simulink model "BatteryEstim3RC_PTBS_v1"  (R2021b)
settings: Solver=ode45  StartTime=0.0  StopTime=3600*100  MaxStep=60  RelTol=1e-3
values from neighbouring files (symbols this model uses):
  CapacityAh = 18.45078888    [CRM_test2.mat]    (also in test_experimentalData.m = p(1,j))
  Em = [45.6901270717 46.4315814068 47.300952453 47.7790115007 48.2148195515 48.8978968293 49.5654324772 50.1873261848 50.9421309599 51.6669224049 52.4024883901 52.7506387312]    [CRM_test2.mat]
  InitialCapVoltage = [0 0 0]    [CRM_test2.mat]
  InitialChargeDeficitAh = 0    [CRM_test2.mat]    (also in test_experimentalData.m = p(2,j)*(1-SOC_0)*CapacityAh)
  R0 = [0.0235875392162 0.0245006787976 0.0256331806458 0.0242487665052 0.028405652821 0.0253523326352 0.028201644819 0.0293858743062 0.0295795385449 0.0307165268423 0.0287680896969 0.030864537146]    [CRM_test2.mat]
  Rx = [0.00541138390772 0.0212793802998 0.00233398938792 0.00525131200495 0.0214750772641 0.0118054508147 0.0052795280688 0.0206172338661 0.0267100492405 0.00529937987512 0.0207294874529 0.0276908855018 ... (36 elements, 3x12)]    [CRM_test2.mat]
  SOC_LUT = [0 0.19733502907 0.397240705949 0.465830267524 0.533618770668 0.604063407396 0.674817039043 0.746547331368 0.819156363357 0.892985414724 0.969511183307 1]    [CRM_test2.mat]
  Tx = [2.08733276285 29.8288343735 111.456817188 2.91727865649 28.0237475362 580.71656132 2.8704763749 27.9272337783 507.228077533 2.8038263246 29.292039832 509.28251447 ... (36 elements, 3x12)]    [CRM_test2.mat]
libraries: autolibbatterycommon x1
settings Model: ModifiedByFormat=The MathWorks, Inc.  Creator=The MathWorks, Inc.  LastModifiedBy=The MathWorks, Inc.
settings SolverCC: AlgebraicLoopSolver=TrustRegion
settings DataIOCC: ExternalInput=[psObj.Time, psObj.Current]  LoadExternalInput=on  SaveOutput=off  DSMLogging=off  SaveTime=off  ReturnWorkspaceOutputs=off
settings DebuggingCC: SFMachineParentedDataDiag=warning  ArithmeticOperatorsInVariantConditions=warning
settings SFSimCC: SimUseLocalCustomCode=off  CustomCodeUndefinedFunction=UseInterfaceOnly
settings RTWCC: RTWUseLocalCustomCode=off
settings CodeAppCC: StateflowObjectComments=on

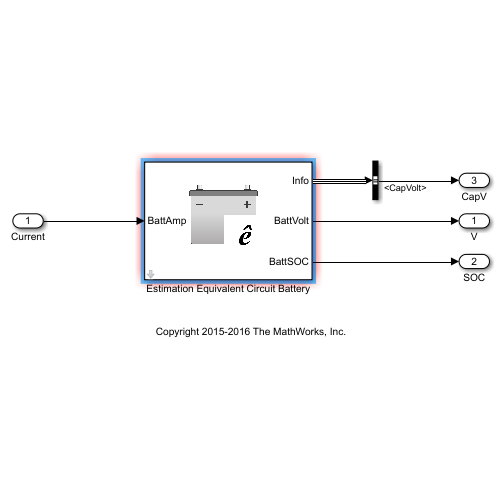
[thumbnail: Simulink's stored preview of the top-level diagram]
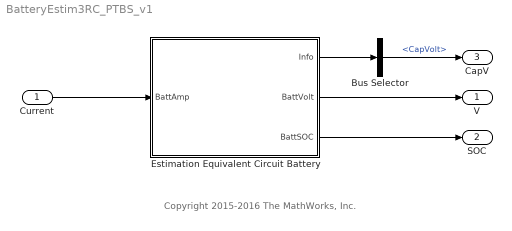
== system BatteryEstim3RC_PTBS_v1 ==
  note: Copyright 2015-2016 The MathWorks, Inc.
  Current : Inport
  Bus Selector : BusSelector  OutputSignals=CapVolt
  Estimation Equivalent Circuit Battery : Subsystem  mask(Estimation Equivalent Circuit Battery){NumRC=4, Em=Em, R0=R0, SOC_BP=SOC_LUT, BattCap=CapacityAh, BattCapInit=CapacityAh-InitialChargeDeficitAh, InitialCapVoltage=InitialCapVoltage, R1=Rx(1,:), C1=Tx(1,:)./Rx(1,:), R2=Rx(2,:), C2=Tx(2,:)./Rx(2,:), R3=Rx(3,:), C3=Tx(3,:)./Rx(3,:), R4=Rx(4,:), C4=Tx(4,:)./Rx(4,:), R5=[0.005 0.005 0.005 0.005 0.005 0.005], C5=[10000 10000 10000 10000 10000 10000], Vu=Inf, Vl=-Inf}
      mask prompts: NumRC "autoblks:autoblkParamEstRcBattery:blkPrm_NumRC"; Em "autoblks:autoblkParamEstRcBattery:blkPrm_Em"; R0 "autoblks:autoblkParamEstRcBattery:blkPrm_R0"; SOC_BP "autoblks:autoblkParamEstRcBattery:blkPrm_SOC_BP"; BattCap "autoblks:autoblkParamEstRcBattery:blkPrm_BattCap"; BattCapInit "autoblks:autoblkParamEstRcBattery:blkPrm_BattCapInit"; InitialCapVoltage "autoblks:autoblkParamEstRcBattery:blkPrm_InitialCapVoltage"; R1 "autoblks:autoblkParamEstRcBattery:blkPrm_R1"; C1 "autoblks:autoblkParamEstRcBattery:blkPrm_C1"; R2 "autoblks:autoblkParamEstRcBattery:blkPrm_R2"; C2 "autoblks:autoblkParamEstRcBattery:blkPrm_C2"; R3 "autoblks:autoblkParamEstRcBattery:blkPrm_R3"; C3 "autoblks:autoblkParamEstRcBattery:blkPrm_C3"; R4 "autoblks:autoblkParamEstRcBattery:blkPrm_R4"; C4 "autoblks:autoblkParamEstRcBattery:blkPrm_C4"; R5 "autoblks:autoblkParamEstRcBattery:blkPrm_R5"; C5 "autoblks:autoblkParamEstRcBattery:blkPrm_C5"; Vu "autoblks:autoblkParamEstRcBattery:blkPrm_Vu"; Vl "autoblks:autoblkParamEstRcBattery:blkPrm_Vl"
      mask help: autoblks:autoblkParamEstRcBattery:blkDesc
      mask init:
      | autoicon('pbbatteryparamest', gcb, 'Initialization');
      mask Help: eval('autoblkshelp(''pbbatteryrcnetworkpe'')');
      mask TypeOptions NumRC: autoblks:autoblkParamEstRcBattery:blkCmb_NumRC1 | autoblks:autoblkParamEstRcBattery:blkCmb_NumRC2 | autoblks:autoblkParamEstRcBattery:blkCmb_NumRC3 | autoblks:autoblkParamEstRcBattery:blkCmb_NumRC4 | autoblks:autoblkParamEstRcBattery:blkCmb_NumRC5
      mask Callback NumRC: autoicon('pbbatteryparamest', gcb, 'NumRCPopup');
      mask DialogControl Container9 Prompt: autoblks:autoblkParamEstRcBattery:blkDlg_Container9
      mask DialogControl NumRC Prompt: Number of series RC pairs:
      mask DialogControl Em Prompt: Open circuit voltage table data, Em [V]:
      mask DialogControl R0 Prompt: Series resistance table data, R0 [Ohm]:
      mask DialogControl SOC_BP Prompt: State of charge breakpoints, SOC_BP []:
      mask DialogControl BattCap Prompt: Battery capacity, BattCap [Ah]:
      mask DialogControl BattCapInit Prompt: Initial battery capacity, BattCapInit [Ah]:
      mask DialogControl InitialCapVoltage Prompt: Initial capacitor voltage, InitialCapVoltage [V]:
      mask DialogControl Container10 Prompt: autoblks:autoblkParamEstRcBattery:blkDlg_Container10
      mask DialogControl R1 Prompt: Network resistance table data, R1 [Ohm]:
      mask DialogControl C1 Prompt: Network capacitance table data, C1 [F]:
      mask DialogControl R2 Prompt: Network resistance table data, R2 [Ohm]:
      mask DialogControl C2 Prompt: Network capacitance table data, C2 [F]:
      mask DialogControl R3 Prompt: Network resistance table data, R3 [Ohm]:
      mask DialogControl C3 Prompt: Network capacitance table data, C3 [F]:
      mask DialogControl R4 Prompt: Network resistance table data, R4 [Ohm]:
      mask DialogControl C4 Prompt: Network capacitance table data, C4 [F]:
      mask DialogControl R5 Prompt: Network resistance table data, R5 [Ohm]:
      mask DialogControl C5 Prompt: Network capacitance table data, C5 [F]:
      mask DialogControl Container7 Prompt: autoblks:autoblkParamEstRcBattery:blkDlg_Container7
      mask DialogControl Vu Prompt: Upper Integrator Voltage Limit, Vu [V]:
      mask DialogControl Vl Prompt: Lower Integrator Voltage Limit, Vl [V]:
      mask Display:
      | IconInfo = autoicon('pbbatteryparamest', gcb, 'DrawCommands');
      | 
      | image(IconInfo.image, IconInfo.position);
      | 
      | for i = 1:numel(IconInfo.lconn)
      |     port_label('lconn', i, IconInfo.lconn{i})
      | end
      | 
      | for j = 1:numel(IconInfo.rconn)
      |     port_label('rconn', j, IconInfo.rconn{j})
      | end
      | 
      | for k = 1:numel(IconInfo.input)
      |     port_label('input', k, IconInfo.input{k})
      | end
      | 
      | for m = 1:numel(IconInfo.output)
      |     port_label('output', m, IconInfo.output{m})
      | end
  V : Outport
  SOC : Outport  Port=2
  CapV : Outport  Port=3
  wires:
  Estimation Equivalent Circuit Battery/1(Info) -> Bus Selector/1
  Bus Selector/1 -> CapV/1  "<CapVolt>"
  Estimation Equivalent Circuit Battery/3(BattSOC) -> SOC/1
  Estimation Equivalent Circuit Battery/2(BattVolt) -> V/1
  Current/1 -> Estimation Equivalent Circuit Battery/1(BattAmp)

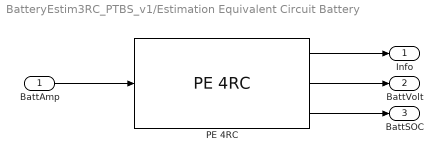
== system BatteryEstim3RC_PTBS_v1/Estimation Equivalent Circuit Battery ==
  BattAmp : Inport
  PE 4RC : autolibbatterycommon/PE 4RC  SystemSampleTime=-1  VariantControl=4  VariantActivationTime=update diagram  Latency=0  AutoFrameSizeCalculation=off
      settings: SourceProductBaseCode=PW
  Info : Outport
  BattVolt : Outport  Port=2
  BattSOC : Outport  Port=3
  wires:
  BattAmp/1 -> PE 4RC/1
  PE 4RC/3 -> BattSOC/1
  PE 4RC/2 -> BattVolt/1
  PE 4RC/1 -> Info/1
